simulink model "DC_Motor_BrakeMode_Ideal"  (R2018a)
settings: Solver=VariableStepAuto  StartTime=0.0  StopTime=10.0  FixedStep=1e-5  RelTol=1e-3
settings Model: Creator=Thomas  LastModifiedBy=Thomas

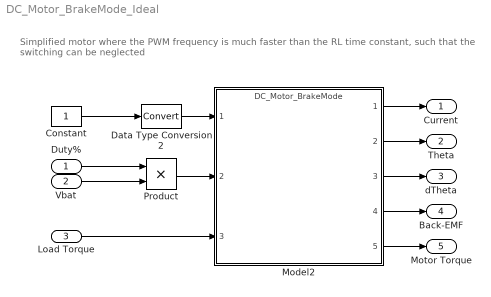
== system DC_Motor_BrakeMode_Ideal ==
  note: Simplified motor where the PWM frequency is much faster than the RL time constant, such that the switching can be neglected
  Duty% : Inport  OutDataTypeStr=double
  Vbat : Inport  Port=2  OutDataTypeStr=double
  Load Torque : Inport  Port=3  OutDataTypeStr=double
  Constant : Constant
  Data Type Conversion2 : DataTypeConversion  RndMeth=Round
  Model2 : ModelReference  ModelNameDialog=DC_Motor_BrakeMode  SimulationMode=Normal  ModelReferenceVersion=1.32
  Product : Product
  Current : Outport
  Theta : Outport  Port=2
  dTheta : Outport  Port=3
  Back-EMF : Outport  Port=4
  Motor Torque : Outport  Port=5
  wires:
  Product/1 -> Model2/2
  Constant/1 -> Data Type Conversion2/1
  Load Torque/1 -> Model2/3
  Model2/1 -> Current/1
  Vbat/1 -> Product/2
  Duty%/1 -> Product/1
  Model2/5 -> Motor Torque/1
  Model2/2 -> Theta/1
  Model2/4 -> Back-EMF/1
  Model2/3 -> dTheta/1
  Data Type Conversion2/1 -> Model2/1
